simulink model "AirRefueling_Platform_Varyingmass"  (R2023a)
settings: Solver=VariableStepAuto  StartTime=0.0  StopTime=100  FixedStep=0.01  RelTol=1e-3  EnableMultiTasking=on
InitFcn:
  | F16_Init
values from neighbouring files (symbols this model uses):
  A_define = A(1:12,1:12)    [F16_Init.m]
  airSpeed = 393.72    [F16_Init.m]
  alpha0 = trimAlpha*180/pi    (= 6.62393794015)    [F16_Init.m]
  altitude = 9843    [F16_Init.m]
  B_define = A(1:12,13:16)    [F16_Init.m]
  b_ref = 30.0    (= 30)    [F16_Init.m]
  C = [ 1,0,0,zeros(1,15) ... (first row only)    [F16_Init.m]
  C2m = [C(1,:) ... (first row only)    [F16_Init.m]
  C_la = [1,0,zeros(1,4)]    [F16_Init.m]
  C_lon = [1,0,zeros(1,4);0,1,zeros(1,4)]    [F16_Init.m]
  Cdr_ = 0.8    [HoseDrogue_Parameter.m]
  d_f_rc = [3.75;0;-1.75]    [F16_Init.m]
  d_pr_cam = d_pr_rc - d_cam_rc    [F16_Init.m]
  d_pr_rc = [7.6;0.50;-2.44]    [F16_Init.m]
  dLEF = 0    [F16_Init.m]
  dtheta10 = zeros(1,N)    [HoseDrogue_Parameter.m]
  dtheta20 = zeros(1,N)    [HoseDrogue_Parameter.m]
  fi_flag = 1    [F16_Init.m]
  height = 3000    [HoseDrogue_Parameter.m]
  Inertia = [9496,0,-982.0;0,55814.0,0;-982.0,0,63100.0]    [F16_Init.m]
  k_reel = 0.5    [HoseDrogue_Parameter.m]
  Kc = [ ... (first row only)    [F16_Init.m]
  kd = 500    [HoseDrogue_Parameter.m]
  Ki = zeros(4,3)    [F16_Init.m]
  Ki_la = -k_la(:,9)    [F16_Init.m]
  Ki_lon = -k_lon(:,9:10)    [F16_Init.m]
  Kp = zeros(4,18)    [F16_Init.m]
  kp_la = Kp_define(3:4,[2,4,6,9,10,12])    [F16_Init.m]
  kp_lon = Kp_define(1:2,[1,3,5,7,8,11])    [F16_Init.m]
  l0 = (length-l1)/(N-1)    (= 1.44444444444)    [HoseDrogue_Parameter.m]
  l1 = 2    [HoseDrogue_Parameter.m]
  l_density = 4.1    [HoseDrogue_Parameter.m]
  m0 = l0*l_density    (= 5.92222222222)    [HoseDrogue_Parameter.m]
  mass = 636.94    [F16_Init.m]
  Mdr = 29.5    [HoseDrogue_Parameter.m]
  N = 10    [HoseDrogue_Parameter.m]    (also in bsp3.m)
  p0_rc = [-30;1;8]    [F16_Init.m]
  Rdr = 0.305    [HoseDrogue_Parameter.m]
  Rl = 0.0336    [HoseDrogue_Parameter.m]
  T_reel_initial = 1610    [HoseDrogue_Parameter.m]
  theta10 = theta1_100    [HoseDrogue_Parameter.m]
  theta20 = theta2_100    [HoseDrogue_Parameter.m]
  trim_ail = 0.00874607850103852    (= 0.00874607850104)    [F16_Init.m]
  trim_control = [trim_thrust;trim_ele;trim_ail;trim_rud]    [F16_Init.m]
  trim_ele = -2.97973164860638    (= -2.97973164861)    [F16_Init.m]
  trim_rud = 0.0680302158182712    (= 0.0680302158183)    [F16_Init.m]
  trim_state = [0;0;0;0;trimAlpha;0;airSpeed;trimAlpha;0;0;0;0]    [F16_Init.m]
  trim_state1 = [trim_state;0;0;0;0;0;0]    [F16_Init.m]
  trim_thrust = 2279.08519954656    (= 2279.08519955)    [F16_Init.m]
  visual_err = [0.07;0.04;-1.21]    [F16_Init.m]
  vt0 = [120;0;0]    [HoseDrogue_Parameter.m]
undefined symbols (not defined in the file or in its folder): A_la_define, A_lon_define, B_la_define, B_lon_define, CC_la, CC_lon, dockingPoint, F, Light, MIL, STD, v_oil
libraries: aerolibconvert2 x13, etargetslib x11, dspnetwork x10, aerolibasang x8, aerolibatmos2 x3, aerolibobsolete x3, simulink x2, aerolibwind2 x2, aerolibadyn x2, sharedtransform x2, aerolibutil x2, vrlib x1
(part 3 of 4)

== system AirRefueling_Platform_Varyingmass/Receiver system/F16 Nonlinear Model/constant mass model/sec_sys_controller ==
  Pri_Obv_States : Inport
  Sec_Obv_States : Inport  Port=2
  " " : Constant  Value=A_lon_define
  "    " : Constant  Value=B_lon_define
  "     " : Constant  Value=A_la_define
  "      " : Constant  Value=B_la_define
  "    1" : Constant  Value=CC_lon
  "    2" : Constant  Value=CC_la
  Demux : Demux
  Gain1 : Gain  Gain=1000
  Lat_Controller : MATLAB Function  TreatAsAtomicUnit=on
  Lon_Controller : MATLAB Function  TreatAsAtomicUnit=on
  Mux : Mux
  Mux13 : Mux  Inputs=2
  Scope : Scope
  Scope1 : Scope
  TrimState1 : Constant  Value=trim_state
  TrimState2 : Constant  Value=trim_state
  Sec_inputs : Outport  VectorParamsAs1DForOutWhenUnconnected=off
  wires:
  Demux/1 -> Gain1/1
  Gain1/1 -> Mux/1
  Mux/1 -> Sec_inputs/1
  Demux/2 -> Mux/2
  Demux/3 -> Mux/3
  Demux/4 -> Mux/4
  Lon_Controller/2(output) -> Mux13/1
  " "/1 -> Lon_Controller/3(A_lon_define)
  "    "/1 -> Lon_Controller/4(B_lon_define)
  "     "/1 -> Lat_Controller/3(A_la_define)
  "      "/1 -> Lat_Controller/4(B_la_define)
  Lat_Controller/1(output) -> Mux13/2
  "    1"/1 -> Lon_Controller/5(CC_lon)
  "    2"/1 -> Lat_Controller/5(CC_la)
  Lon_Controller/1(s) -> Scope/1
  Lat_Controller/2(s) -> Scope1/1
  Mux13/1 -> Demux/1
  Sec_Obv_States/1 -> Lat_Controller/2(Sec_States), Lon_Controller/1(Sec_States)
  Pri_Obv_States/1 -> Lat_Controller/1(Pri_States), Lon_Controller/2(Pri_States)
  TrimState1/1 -> Lat_Controller/6(trim_states)
  TrimState2/1 -> Lon_Controller/6(trim_states)

== system AirRefueling_Platform_Varyingmass/Receiver system/F16 Nonlinear Model/Variable Mass Model/Aerodynamic Coefficients1/Leading Edge Flap ==
  note: see NASA Technical Paper 1538, p34
  note: Initialize LF_state with -alpha0 value in degrees!!!!
  alpha : Inport
  qbar/ps : Inport  Port=2
  Gain : Gain  Gain=2  SaturateOnIntegerOverflow=on  OutDataTypeStr=Inherit: Same as input  ParamDataTypeStr=Inherit: Same as input
  Gain1 : Gain  Gain=7.25  SaturateOnIntegerOverflow=on  OutDataTypeStr=Inherit: Same as input  ParamDataTypeStr=Inherit: Same as input
  Gain2 : Gain  Gain=1.38  SaturateOnIntegerOverflow=on  OutDataTypeStr=Inherit: Same as input  ParamDataTypeStr=Inherit: Same as input
  LEF Actuator : Subsystem
  LF_state : Integrator  InitialCondition=-alpha0
  Sum : Sum  Inputs=-|+|+  InputSameDT=on  SaturateOnIntegerOverflow=on  OutDataTypeStr=Inherit: Same as first input
  Sum1 : Sum  Inputs=|+-  InputSameDT=on  SaturateOnIntegerOverflow=on  OutDataTypeStr=Inherit: Same as first input
  Sum2 : Sum  Inputs=++|  InputSameDT=on  SaturateOnIntegerOverflow=on  OutDataTypeStr=Inherit: Same as first input
  coeff1 : Constant  Value=1.45
  lef Saturation : Saturate  UpperLimit=25  LowerLimit=0
  r2d6 : Gain  Gain=9.05  SaturateOnIntegerOverflow=on  OutDataTypeStr=Inherit: Same as input  ParamDataTypeStr=Inherit: Same as input
  delta_lef (deg) : Outport
  wires:
  Sum1/1 -> Gain1/1
  Gain1/1 -> LF_state/1
  Gain/1 -> Sum2/1
  Gain2/1 -> Sum/2
  coeff1/1 -> Sum/3
  Sum2/1 -> Sum1/2, Gain2/1
  LF_state/1 -> Sum2/2
  alpha/1 -> Sum1/1, Gain/1
  qbar/ps/1 -> r2d6/1
  r2d6/1 -> Sum/1
  lef Saturation/1 -> delta_lef (deg)/1
  Sum/1 -> LEF Actuator/1(dlef)
  LEF Actuator/1(LEF) -> lef Saturation/1

== system AirRefueling_Platform_Varyingmass/Receiver system/F16 Nonlinear Model/Variable Mass Model/actuator1/Aileron Actuator ==
  delta_a : Inport
  Command Saturation : Saturate  UpperLimit=21.5  LowerLimit=-21.5
  Gain : Gain  Gain=20.2  SaturateOnIntegerOverflow=on  OutDataTypeStr=Inherit: Same as input  ParamDataTypeStr=Inherit: Same as input
  "Integrator " : Integrator  InitialCondition=trim_ail  UpperSaturationLimit=21.5  LowerSaturationLimit=-21.5
  Rate Saturation : Saturate  UpperLimit=80  LowerLimit=-80
  Sum : Sum  Inputs=|+-  InputSameDT=on  SaturateOnIntegerOverflow=on  OutDataTypeStr=Inherit: Same as first input
  ail : Outport
  wires:
  delta_a/1 -> Command Saturation/1
  "Integrator "/1 -> ail/1, Sum/2
  Sum/1 -> Gain/1
  Gain/1 -> Rate Saturation/1
  Command Saturation/1 -> Sum/1
  Rate Saturation/1 -> "Integrator "/1

== system AirRefueling_Platform_Varyingmass/Receiver system/F16 Nonlinear Model/Variable Mass Model/actuator1/Elevator Actuator ==
  delta_e : Inport
  Command Saturation : Saturate  UpperLimit=25  LowerLimit=-25
  Gain : Gain  Gain=20.2  SaturateOnIntegerOverflow=on  OutDataTypeStr=Inherit: Same as input  ParamDataTypeStr=Inherit: Same as input
  "Integrator " : Integrator  InitialCondition=trim_ele  UpperSaturationLimit=25  LowerSaturationLimit=-25
  Rate Saturation : Saturate  UpperLimit=60  LowerLimit=-60
  Sum : Sum  Inputs=|+-  InputSameDT=on  SaturateOnIntegerOverflow=on  OutDataTypeStr=Inherit: Same as first input
  el : Outport
  wires:
  delta_e/1 -> Command Saturation/1
  Command Saturation/1 -> Sum/1
  Sum/1 -> Gain/1
  Gain/1 -> Rate Saturation/1
  "Integrator "/1 -> el/1, Sum/2
  Rate Saturation/1 -> "Integrator "/1

== system AirRefueling_Platform_Varyingmass/Receiver system/F16 Nonlinear Model/Variable Mass Model/actuator1/Rudder Actuator ==
  delta_r : Inport
  Command Saturation : Saturate  UpperLimit=30  LowerLimit=-30
  Gain : Gain  Gain=20.2  SaturateOnIntegerOverflow=on  OutDataTypeStr=Inherit: Same as input  ParamDataTypeStr=Inherit: Same as input
  "Integrator " : Integrator  InitialCondition=trim_rud  UpperSaturationLimit=30  LowerSaturationLimit=-30
  Rate Saturation : Saturate  UpperLimit=120  LowerLimit=-120
  Sum : Sum  Inputs=|+-  InputSameDT=on  SaturateOnIntegerOverflow=on  OutDataTypeStr=Inherit: Same as first input
  rud : Outport
  wires:
  "Integrator "/1 -> rud/1, Sum/2
  Sum/1 -> Gain/1
  delta_r/1 -> Command Saturation/1
  Rate Saturation/1 -> "Integrator "/1
  Gain/1 -> Rate Saturation/1
  Command Saturation/1 -> Sum/1

== system AirRefueling_Platform_Varyingmass/Receiver system/F16 Nonlinear Model/Variable Mass Model/actuator1/Thrust Model ==
  delta_t : Inport
  Command Saturation : Saturate  UpperLimit=19000  LowerLimit=1000
  Gain : Gain  SaturateOnIntegerOverflow=on  OutDataTypeStr=Inherit: Same as input  ParamDataTypeStr=Inherit: Same as input
  "Integrator " : Integrator  InitialCondition=trim_thrust  UpperSaturationLimit=30  LowerSaturationLimit=-30
  Rate Saturation : Saturate  UpperLimit=10000  LowerLimit=-10000
  Sum : Sum  Inputs=|+-  InputSameDT=on  SaturateOnIntegerOverflow=on  OutDataTypeStr=Inherit: Same as first input
  T : Outport
  wires:
  delta_t/1 -> Command Saturation/1
  Gain/1 -> Rate Saturation/1
  "Integrator "/1 -> T/1, Sum/2
  Command Saturation/1 -> Sum/1
  Sum/1 -> Gain/1
  Rate Saturation/1 -> "Integrator "/1

== system AirRefueling_Platform_Varyingmass/Receiver system/F16 Nonlinear Model/constant mass model/F-16/Adding Wind Disturbance ==
  Speed of Sound : Inport
  Air Density : Inport  Port=2
  Wind Velocity : Inport  Port=3  PortDimensions=3
  Wind Angular Rates : Inport  Port=4  PortDimensions=3
  Vb : Inport  Port=5  PortDimensions=3
  p,q,r : Inport  Port=6  PortDimensions=3
  Display : Display
  Dynamic Pressure : aerolibasang/Dynamic Pressure
  "Incidence, Sideslip & Airspeed" : aerolibasang/Incidence, Sideslip, & Airspeed
  Mach Number : aerolibasang/Mach Number
  Mux : Mux  Inputs=2
  Sum : Sum  Inputs=|+-  InputSameDT=on  SaturateOnIntegerOverflow=on  OutDataTypeStr=Inherit: Same as first input
  Sum1 : Sum  Inputs=|++  InputSameDT=on  SaturateOnIntegerOverflow=on  OutDataTypeStr=Inherit: Same as first input
  qbar : Outport  InitialOutput=0
  "p,q,r " : Outport  Port=2
  V : Outport  Port=3
  Mach : Outport  Port=4
  Incid : Outport  Port=5
  wires:
  "Incidence, Sideslip & Airspeed"/3 -> V/1
  Dynamic Pressure/1 -> qbar/1
  Air Density/1 -> Dynamic Pressure/2
  Mach Number/1 -> Mach/1
  Sum/1 -> Dynamic Pressure/1, Mach Number/1, "Incidence, Sideslip & Airspeed"/1
  Vb/1 -> Display/1, Sum/1
  Speed of Sound/1 -> Mach Number/2
  Wind Velocity/1 -> Sum/2
  "Incidence, Sideslip & Airspeed"/2 -> Mux/2  "Beta"
  Mux/1 -> Incid/1
  "Incidence, Sideslip & Airspeed"/1 -> Mux/1  "Alpha"
  p,q,r/1 -> Sum1/1
  Wind Angular Rates/1 -> Sum1/2
  Sum1/1 -> "p,q,r "/1

== system AirRefueling_Platform_Varyingmass/Receiver system/F16 Nonlinear Model/constant mass model/F-16/Aerodynamic Coefficients ==
  Actuators : Inport
  Incid : Inport  Port=2
  Mach : Inport  Port=3
  V : Inport  Port=4
  p,q,r : Inport  Port=5
  qbar/ps : Inport  Port=6
  Angle Conversion : aerolibconvert2/Angle Conversion  IU=rad  OU=deg
  Display : Display
  Interpreted MATLAB Function : MATLABFcn  MATLABFcn=F16Coef1  OutputDimensions=6
  Leading Edge Flap : Subsystem
  Mux : Mux  Inputs=6
  Terminator2 : Terminator
  alpha : Selector  InputPortWidth=2  IndexOptions=Index vector (dialog)  Indices=1  OutputSizes=1
  flag : Constant  Value=fi_flag
  Coeff : Outport  InitialOutput=0
  wires:
  Angle Conversion/1 -> alpha/1, Mux/2
  Incid/1 -> Angle Conversion/1
  qbar/ps/1 -> Leading Edge Flap/2(qbar/ps)
  alpha/1 -> Leading Edge Flap/1(alpha)
  V/1 -> Display/1, Mux/1
  p,q,r/1 -> Mux/3
  Actuators/1 -> Mux/4
  flag/1 -> Mux/5
  Mach/1 -> Terminator2/1
  Interpreted MATLAB Function/1 -> Coeff/1
  Mux/1 -> Interpreted MATLAB Function/1
  Leading Edge Flap/1(delta_lef (deg)) -> Mux/6

== system AirRefueling_Platform_Varyingmass/Receiver system/F16 Nonlinear Model/constant mass model/F-16/Environment Models ==
  Xe : Inport  PortDimensions=3
  DCM : Inport  Port=2
  COESA Atmosphere Model : aerolibatmos2/COESA Atmosphere Model  units=English (Velocity in ft/s)  spec=1976 COESA-extended U.S. Standard Atmosphere  model=Profile  profile_var=High temperature  profile_percent=10%  profile_alt=5 km (16404 ft)  envelope_var=High temperature  envelope_percent=1%  action=None
  Display : Display
  Display1 : Display
  Gravity in Earth Axes : Gain  Gain=mass  SaturateOnIntegerOverflow=on  OutDataTypeStr=Inherit: Same as input  ParamDataTypeStr=Inherit: Same as input
  Height : Selector  InputPortWidth=3  IndexOptions=Index vector (dialog)  Indices=[3]  OutputSizes=1
  Inertial to Body : Product  Multiplication=Matrix(*)  InputSameDT=on  SaturateOnIntegerOverflow=on  OutDataTypeStr=Inherit: Same as first input
  Latitude : Constant  Value=0
  Mux : Mux  Inputs=3
  Product6 : Product  Inputs=**  InputSameDT=on  SaturateOnIntegerOverflow=on  OutDataTypeStr=Inherit: Same as first input
  Reshape : Reshape
  Terminator : Terminator
  "WGS84 Gravity Model " : aerolibobsolete/WGS84 Gravity Model   model=WGS84 Taylor Series  units=English  no_atmos=on  precessing=on  jd_loc=off  month=October  day=10  year=2004  no_centrifugal=on  action=None
  r2d5 : Gain  Gain=1715  SaturateOnIntegerOverflow=on  OutDataTypeStr=Inherit: Same as input  ParamDataTypeStr=Inherit: Same as input
  z-->h : Abs
  Fg : Outport  InitialOutput=0
  Speed of Sound : Outport  Port=2  InitialOutput=0
  Air Density : Outport  Port=3  InitialOutput=0
  PS : Outport  Port=4
  wires:
  Reshape/1 -> Inertial to Body/2
  Mux/1 -> "WGS84 Gravity Model "/1
  z-->h/1 -> Mux/3, COESA Atmosphere Model/1
  COESA Atmosphere Model/2 -> Speed of Sound/1
  COESA Atmosphere Model/3 -> Terminator/1
  Height/1 -> z-->h/1
  Xe/1 -> Height/1
  Latitude/1 -> Mux/2, Mux/1
  "WGS84 Gravity Model "/1 -> Gravity in Earth Axes/1
  Gravity in Earth Axes/1 -> Reshape/1
  DCM/1 -> Inertial to Body/1
  Inertial to Body/1 -> Display1/1, Fg/1
  COESA Atmosphere Model/4 -> Product6/2, Air Density/1
  COESA Atmosphere Model/1 -> r2d5/1
  Product6/1 -> Display/1, PS/1
  r2d5/1 -> Product6/1

== system AirRefueling_Platform_Varyingmass/Receiver system/F16 Nonlinear Model/constant mass model/F-16/Forces and Moments ==
  Coeff : Inport
  Thrust : Inport  Port=2
  qbar : Inport  Port=3
  "Aerodynamic Forces and Moments " : aerolibadyn/Aerodynamic Forces and Moments   inputAxes=Body  outputForceAxes=Body  outputMomentAxes=Body  S=S_ref  b=b_ref  cbar=d_ref
  Center of Gravity : Constant  Value=[-0 0 0]
  Center of Pressure : Constant  Value=[-0 0 0]
  Sum : Sum  Inputs=++|  InputSameDT=on  SaturateOnIntegerOverflow=on  OutDataTypeStr=Inherit: Same as first input
  X,Y,Z : Outport  InitialOutput=0
  LMN : Outport  Port=2  InitialOutput=0
  wires:
  Center of Pressure/1 -> "Aerodynamic Forces and Moments "/4
  Center of Gravity/1 -> "Aerodynamic Forces and Moments "/3
  "Aerodynamic Forces and Moments "/1 -> Sum/2
  "Aerodynamic Forces and Moments "/2 -> LMN/1
  Sum/1 -> X,Y,Z/1
  Thrust/1 -> Sum/1
  qbar/1 -> "Aerodynamic Forces and Moments "/2
  Coeff/1 -> "Aerodynamic Forces and Moments "/1

== system AirRefueling_Platform_Varyingmass/Receiver system/F16 Nonlinear Model/constant mass model/F-16/Subsystem ==
  <Eular(rad)> : Inport
  DCM : Inport  Port=2
  Ve : Inport  Port=3
  X_relative : Inport  Port=4
  pqr : Inport  Port=5
  Constant1 : Constant  Value=mass
  Constant5 : Constant  Value=dockingPoint
  Direction Cosine Matrix to Quaternions : sharedtransform/Direction Cosine Matrix  to Quaternions  aMode=aMode  action=None  tolerance=eps(2)
  Direction Cosine Matrix to Quaternions1 : sharedtransform/Direction Cosine Matrix  to Quaternions  aMode=aMode  action=None  tolerance=eps(2)
  Euler to DCM : aerolibtransform2/Wind Angles to  Direction Cosine Matrix
  Ground Model : MATLAB Function  TreatAsAtomicUnit=on
  Length Conversion : aerolibconvert2/Length Conversion  IU=ft  OU=m
  OnGroundFaceup : MATLAB Function  TreatAsAtomicUnit=on
  Product1 : Product  Multiplication=Matrix(*)
  Quaternion Inverse : aerolibutil/Quaternion Inverse
  Quaternion Multiplication : aerolibutil/Quaternion Multiplication
  Scope : Scope
  Scope1 : Scope
  Scope2 : Scope
  Sum : Sum  Inputs=|-+
  F1 : Outport
  M1 : Outport  Port=2
  wires:
  Length Conversion/1 -> Sum/1, Ground Model/3(X_relative)
  Direction Cosine Matrix to Quaternions/1 -> Quaternion Multiplication/2
  Constant5/1 -> Sum/2, Ground Model/6(dockingPoint)
  pqr/1 -> Ground Model/2(wb)
  Euler to DCM/1 -> Direction Cosine Matrix to Quaternions1/1
  DCM/1 -> Product1/1, Direction Cosine Matrix to Quaternions/1
  Ground Model/1(F1) -> Scope/1, Product1/2
  Quaternion Inverse/1 -> Quaternion Multiplication/1
  <Eular(rad)>/1 -> OnGroundFaceup/1(EulerAng)
  OnGroundFaceup/1(y) -> Euler to DCM/1
  X_relative/1 -> Length Conversion/1
  Direction Cosine Matrix to Quaternions1/1 -> Quaternion Inverse/1
  Product1/1 -> Scope1/1, F1/1
  Quaternion Multiplication/1 -> Ground Model/5(Quet)
  Ground Model/2(M1) -> M1/1
  Ve/1 -> Ground Model/4(Ve)
  Sum/1 -> Scope2/1
  Constant1/1 -> Ground Model/1(mass)

== system AirRefueling_Platform_Varyingmass/Receiver system/F16 Nonlinear Model/constant mass model/F-16/actuator ==
  u : Inport
  Aileron Actuator : Subsystem
  Demux : Demux
  Elevator Actuator : Subsystem
  Mux : Mux
  Mux1 : Mux  Inputs=3
  Mux2 : Mux  Inputs=3
  Rudder Actuator : Subsystem
  Thrust Model : Subsystem
  Ty : Constant  Value=0
  Tz : Constant  Value=0
  Ang : Outport
  T : Outport  Port=2
  uc : Outport  Port=3
  wires:
  u/1 -> Demux/1
  Mux2/1 -> Ang/1
  Thrust Model/1(T) -> Mux/1, Mux1/1  "Tx"
  Ty/1 -> Mux1/2
  Tz/1 -> Mux1/3
  Mux1/1 -> T/1
  Mux/1 -> uc/1
  Demux/1 -> Thrust Model/1(delta_t)
  Elevator Actuator/1(el) -> Mux2/1, Mux/2  "el"
  Aileron Actuator/1(ail) -> Mux2/2, Mux/3  "ail"
  Rudder Actuator/1(rud) -> Mux2/3, Mux/4  "rud"
  Demux/2 -> Elevator Actuator/1(delta_e)
  Demux/3 -> Aileron Actuator/1(delta_a)
  Demux/4 -> Rudder Actuator/1(delta_r)

== system AirRefueling_Platform_Varyingmass/Receiver system/F16 Nonlinear Model/Variable Mass Model/Aerodynamic Coefficients1/Leading Edge Flap/LEF Actuator ==
  dlef : Inport
  Command Saturation : Saturate  UpperLimit=25  LowerLimit=0
  Gain3 : Gain  Gain=1/0.136  SaturateOnIntegerOverflow=on  OutDataTypeStr=Inherit: Same as input  ParamDataTypeStr=Inherit: Same as input
  "Integrator " : Integrator  InitialCondition=dLEF  UpperSaturationLimit=21.5  LowerSaturationLimit=-21.5
  Rate Saturation : Saturate  UpperLimit=25  LowerLimit=-25
  Sum3 : Sum  Inputs=|+-  InputSameDT=on  SaturateOnIntegerOverflow=on  OutDataTypeStr=Inherit: Same as first input
  LEF : Outport
  wires:
  Gain3/1 -> Rate Saturation/1
  Rate Saturation/1 -> "Integrator "/1
  "Integrator "/1 -> LEF/1, Sum3/2
  Sum3/1 -> Gain3/1
  dlef/1 -> Command Saturation/1
  Command Saturation/1 -> Sum3/1

== system AirRefueling_Platform_Varyingmass/Receiver system/F16 Nonlinear Model/constant mass model/F-16/Aerodynamic Coefficients/Leading Edge Flap ==
  note: see NASA Technical Paper 1538, p34
  note: Initialize LF_state with -alpha0 value in degrees!!!!
  alpha : Inport
  qbar/ps : Inport  Port=2
  Gain : Gain  Gain=2  SaturateOnIntegerOverflow=on  OutDataTypeStr=Inherit: Same as input  ParamDataTypeStr=Inherit: Same as input
  Gain1 : Gain  Gain=7.25  SaturateOnIntegerOverflow=on  OutDataTypeStr=Inherit: Same as input  ParamDataTypeStr=Inherit: Same as input
  Gain2 : Gain  Gain=1.38  SaturateOnIntegerOverflow=on  OutDataTypeStr=Inherit: Same as input  ParamDataTypeStr=Inherit: Same as input
  LEF Actuator : Subsystem
  LF_state : Integrator  InitialCondition=-alpha0
  Sum : Sum  Inputs=-|+|+  InputSameDT=on  SaturateOnIntegerOverflow=on  OutDataTypeStr=Inherit: Same as first input
  Sum1 : Sum  Inputs=|+-  InputSameDT=on  SaturateOnIntegerOverflow=on  OutDataTypeStr=Inherit: Same as first input
  Sum2 : Sum  Inputs=++|  InputSameDT=on  SaturateOnIntegerOverflow=on  OutDataTypeStr=Inherit: Same as first input
  coeff1 : Constant  Value=1.45
  lef Saturation : Saturate  UpperLimit=25  LowerLimit=0
  r2d6 : Gain  Gain=9.05  SaturateOnIntegerOverflow=on  OutDataTypeStr=Inherit: Same as input  ParamDataTypeStr=Inherit: Same as input
  delta_lef (deg) : Outport
  wires:
  Sum1/1 -> Gain1/1
  Gain1/1 -> LF_state/1
  Gain/1 -> Sum2/1
  Gain2/1 -> Sum/2
  coeff1/1 -> Sum/3
  Sum2/1 -> Sum1/2, Gain2/1
  LF_state/1 -> Sum2/2
  alpha/1 -> Sum1/1, Gain/1
  qbar/ps/1 -> r2d6/1
  r2d6/1 -> Sum/1
  lef Saturation/1 -> delta_lef (deg)/1
  Sum/1 -> LEF Actuator/1(dlef)
  LEF Actuator/1(LEF) -> lef Saturation/1

== system AirRefueling_Platform_Varyingmass/Receiver system/F16 Nonlinear Model/constant mass model/F-16/actuator/Aileron Actuator ==
  delta_a : Inport
  Command Saturation : Saturate  UpperLimit=21.5  LowerLimit=-21.5
  Gain : Gain  Gain=20.2  SaturateOnIntegerOverflow=on  OutDataTypeStr=Inherit: Same as input  ParamDataTypeStr=Inherit: Same as input
  "Integrator " : Integrator  InitialCondition=trim_ail  UpperSaturationLimit=21.5  LowerSaturationLimit=-21.5
  Rate Saturation : Saturate  UpperLimit=80  LowerLimit=-80
  Sum : Sum  Inputs=|+-  InputSameDT=on  SaturateOnIntegerOverflow=on  OutDataTypeStr=Inherit: Same as first input
  ail : Outport
  wires:
  delta_a/1 -> Command Saturation/1
  "Integrator "/1 -> ail/1, Sum/2
  Sum/1 -> Gain/1
  Gain/1 -> Rate Saturation/1
  Command Saturation/1 -> Sum/1
  Rate Saturation/1 -> "Integrator "/1

== system AirRefueling_Platform_Varyingmass/Receiver system/F16 Nonlinear Model/constant mass model/F-16/actuator/Elevator Actuator ==
  delta_e : Inport
  Command Saturation : Saturate  UpperLimit=25  LowerLimit=-25
  Gain : Gain  Gain=20.2  SaturateOnIntegerOverflow=on  OutDataTypeStr=Inherit: Same as input  ParamDataTypeStr=Inherit: Same as input
  "Integrator " : Integrator  InitialCondition=trim_ele  UpperSaturationLimit=25  LowerSaturationLimit=-25
  Rate Saturation : Saturate  UpperLimit=60  LowerLimit=-60
  Sum : Sum  Inputs=|+-  InputSameDT=on  SaturateOnIntegerOverflow=on  OutDataTypeStr=Inherit: Same as first input
  el : Outport
  wires:
  delta_e/1 -> Command Saturation/1
  Command Saturation/1 -> Sum/1
  Sum/1 -> Gain/1
  Gain/1 -> Rate Saturation/1
  "Integrator "/1 -> el/1, Sum/2
  Rate Saturation/1 -> "Integrator "/1

== system AirRefueling_Platform_Varyingmass/Receiver system/F16 Nonlinear Model/constant mass model/F-16/actuator/Rudder Actuator ==
  delta_r : Inport
  Command Saturation : Saturate  UpperLimit=30  LowerLimit=-30
  Gain : Gain  Gain=20.2  SaturateOnIntegerOverflow=on  OutDataTypeStr=Inherit: Same as input  ParamDataTypeStr=Inherit: Same as input
  "Integrator " : Integrator  InitialCondition=trim_rud  UpperSaturationLimit=30  LowerSaturationLimit=-30
  Rate Saturation : Saturate  UpperLimit=120  LowerLimit=-120
  Sum : Sum  Inputs=|+-  InputSameDT=on  SaturateOnIntegerOverflow=on  OutDataTypeStr=Inherit: Same as first input
  rud : Outport
  wires:
  "Integrator "/1 -> rud/1, Sum/2
  Sum/1 -> Gain/1
  delta_r/1 -> Command Saturation/1
  Rate Saturation/1 -> "Integrator "/1
  Gain/1 -> Rate Saturation/1
  Command Saturation/1 -> Sum/1

== system AirRefueling_Platform_Varyingmass/Receiver system/F16 Nonlinear Model/constant mass model/F-16/actuator/Thrust Model ==
  delta_t : Inport
  Command Saturation : Saturate  UpperLimit=19000  LowerLimit=1000
  Gain : Gain  SaturateOnIntegerOverflow=on  OutDataTypeStr=Inherit: Same as input  ParamDataTypeStr=Inherit: Same as input
  "Integrator " : Integrator  InitialCondition=trim_thrust  UpperSaturationLimit=30  LowerSaturationLimit=-30
  Rate Saturation : Saturate  UpperLimit=10000  LowerLimit=-10000
  Sum : Sum  Inputs=|+-  InputSameDT=on  SaturateOnIntegerOverflow=on  OutDataTypeStr=Inherit: Same as first input
  T : Outport
  wires:
  delta_t/1 -> Command Saturation/1
  Gain/1 -> Rate Saturation/1
  "Integrator "/1 -> T/1, Sum/2
  Command Saturation/1 -> Sum/1
  Sum/1 -> Gain/1
  Rate Saturation/1 -> "Integrator "/1

== system AirRefueling_Platform_Varyingmass/Receiver system/F16 Nonlinear Model/constant mass model/F-16/Aerodynamic Coefficients/Leading Edge Flap/LEF Actuator ==
  dlef : Inport
  Command Saturation : Saturate  UpperLimit=25  LowerLimit=0
  Gain3 : Gain  Gain=1/0.136  SaturateOnIntegerOverflow=on  OutDataTypeStr=Inherit: Same as input  ParamDataTypeStr=Inherit: Same as input
  "Integrator " : Integrator  InitialCondition=dLEF  UpperSaturationLimit=21.5  LowerSaturationLimit=-21.5
  Rate Saturation : Saturate  UpperLimit=25  LowerLimit=-25
  Sum3 : Sum  Inputs=|+-  InputSameDT=on  SaturateOnIntegerOverflow=on  OutDataTypeStr=Inherit: Same as first input
  LEF : Outport
  wires:
  Gain3/1 -> Rate Saturation/1
  Rate Saturation/1 -> "Integrator "/1
  "Integrator "/1 -> LEF/1, Sum3/2
  Sum3/1 -> Gain3/1
  dlef/1 -> Command Saturation/1
  Command Saturation/1 -> Sum3/1

== matlab function AirRefueling_Platform_Varyingmass/SimToVR2 ==
  data: PosPr1 input; PosTb1 input; y output
function y = SimToVR(PosPr1,PosTb1)
%#codegen

%%函数名：SimToVR
%%用途  ：将软管锥套坐标输出转换为VR输入
%%输入  ：PosPr - 受油机椎管坐标， PlsTb - 软管坐标数据
%%输出  ：VrPos - 软管和受油机VR位置，VrAngle - 旋转角度输出
%%作者  ：戴训华
%%时间  ：2014/3/19

PosPr = PosPr1(1:3);
AttitudeRecei = [0;-0;0+0.115609];

PosTb = PosTb1(1:60);

VrAngle = zeros(22*4,1);
VrPos = zeros(22*3,1);


for j = 1:21                        %前20为软管坐标数据，后1为软管平滑过渡处理
    if j == 1
        pX = [0, 0, 0]';            %软管起点
        pY = PosTb(3*j-2:3*j);      %软杆终点
    elseif j == 21                  %多加一段杆，做过渡
        pX = PosTb(3*j-5:3*j-3);
        pY = [PosTb(3*j-5)-0.7163*cos(8/180*pi),PosTb(3*j-4),PosTb(3*j-3)+0.7163*sin(8/180*pi)]'+[0;-0.2;0];
    else
        pX = PosTb(3*j-5:3*j-3);
        pY = PosTb(3*j-2:3*j); 
    end
    
    pZ = (pX + pY)/2;               %中点坐标
    pZ = pZ * 8/3;                  %到VR中比例的缩放

    vAxis = [0,0,-1]';               %水平轴
    vTb = pY - pX;                  %杆的方向
    
    axis1 = null([vAxis';vTb']);%获取垂直向量
    vRot = axis1(:,1)';             %得到旋转轴
    
    if vRot(2) < 0
        vRot = -vRot;
    end
    
    VrAngle(4*j-3:4*j-1) = [vRot(1),vRot(3),vRot(2)]';
    VrAngle(4*j) = acos(vAxis'*vTb / sqrt(vAxis'*vAxis * vTb'*vTb));
    
    VrPos(3*j-2:3*j) = [pZ(1),-pZ(3),pZ(2)]';
end
%y = u;
VrAngle(81:84)=VrAngle(81:84)+[0.2714;0;0;0]; %微调锥套姿态
VrPos(61:63)=VrPos(61:63)+[0;0.00;0.25];      %微调锥套位置

VrAngle(85:88)=[AttitudeRecei(1);AttitudeRecei(2);AttitudeRecei(3);norm(AttitudeRecei)];
pZ = PosPr+[0 0-0.1 0-0.1]';
pZ = pZ * 8/3;
VrPos(3*22-2:3*22) = [pZ(1),-pZ(3),pZ(2)]';

y = [VrAngle;VrPos];

== matlab function AirRefueling_Platform_Varyingmass/Hose-drogue system/DRdynamics/HDU/MATLAB Function2 ==
  data: l_1 input; T0 input; Tt output size=1; t input; dl input; l1 parameter; k_reel parameter; kd parameter
function Tt = fcn(l_1,T0,t,dl, l1,k_reel,kd)
Treel = T0*(l_1/l1)^k_reel;
Tt = t - Treel - kd*dl;

== matlab function AirRefueling_Platform_Varyingmass/Receiver system/F16 Nonlinear Model/constant mass model/Observer/Nonlinear Term ==
  data: trimed_states input; y output; A_la_define input; A_lon_define input; trim_states input
function y = fcn(trimed_states,A_la_define,A_lon_define,trim_states)
%% 原状态值（配平前的）
ori_states = trimed_states + trim_states;
phi_ori = ori_states(4);
theta_ori = ori_states(5);
psi_ori = ori_states(6);
Vr_ori = ori_states(7);
alpha_ori = ori_states(8);
beta_ori = ori_states(9);
p_ori = ori_states(10);
q_ori = ori_states(11);
r_ori = ori_states(12);

ug_ori = Vr_ori * cos(alpha_ori) * cos(beta_ori);
vg_ori = Vr_ori * sin(beta_ori);
wg_ori = Vr_ori * sin(alpha_ori) * cos(beta_ori);

xg_ori = ug_ori*cos(theta_ori)*cos(psi_ori) + vg_ori*(sin(phi_ori)*sin(theta_ori)*cos(psi_ori)-cos(phi_ori)*sin(psi_ori)) ...
     + wg_ori*(sin(phi_ori)*sin(psi_ori)+cos(phi_ori)*sin(theta_ori)*cos(psi_ori));
yg_ori = ug_ori*cos(theta_ori)*sin(psi_ori) + vg_ori*(sin(phi_ori)*sin(theta_ori)*sin(psi_ori)+cos(phi_ori)*cos(psi_ori)) ...
     + wg_ori*(-sin(phi_ori)*cos(psi_ori) + cos(phi_ori)*sin(theta_ori)*sin(psi_ori));
hg_ori = ug_ori*sin(theta_ori) - vg_ori*sin(phi_ori)*cos(theta_ori) - wg_ori*cos(phi_ori)*cos(theta_ori);
%% 差状态值（配平后的）
phi_trimed = trimed_states(4);
theta_trimed = trimed_states(5);
psi_trimed = trimed_states(6);
Vr_trimed = trimed_states(7);
alpha_trimed = trimed_states(8);
beta_trimed = trimed_states(9);
p_trimed = trimed_states(10);
q_trimed = trimed_states(11);
r_trimed = trimed_states(12);

% x_nonlinear = Vr_ori * cos(theta_ori - alpha_ori) - A_lon_define(1,3) * theta_trimed - Vr_ori;
% y_nonlinear = Vr_ori * cos(theta_ori - alpha_ori) * sin(psi_ori + beta_ori) - A_la_define(1,2) * phi_trimed - A_la_define(1,3) * psi_trimed - A_la_define(1,4) * beta_trimed;
% h_nonlinear = hg_ori  - A_lon_define(2,3) * (theta_trimed - alpha_trimed);

x_nonlinear = Vr_ori * cos(theta_ori - alpha_ori) - trim_states(7)*cos(trim_states(5)-trim_states(8)) - A_lon_define(1,3) * theta_trimed - Vr_trimed;
y_nonlinear = yg_ori - A_la_define(1,2) * phi_trimed - A_la_define(1,3) * psi_trimed - A_la_define(1,4) * beta_trimed;
h_nonlinear = Vr_ori * sin(theta_ori - alpha_ori) - A_lon_define(2,3) * (theta_trimed - alpha_trimed);
psi_nonlinear = (q_ori*sin(phi_ori) + r_ori*cos(phi_ori))/cos(theta_ori) - A_la_define(3,6) * r_trimed;  % psi
phi_nonlinear = p_ori + tan(theta_ori)*(q_ori*sin(phi_ori)+r_ori*cos(phi_ori)) - A_la_define(2,5) * p_trimed - A_la_define(2,6) * r_trimed;  % phi


y = [x_nonlinear; y_nonlinear; h_nonlinear; phi_nonlinear; 0; psi_nonlinear; 0;0;0;0;0;0];

== matlab function AirRefueling_Platform_Varyingmass/SimToUE ==
  data: y output; PosRc input; PosTb1 input; Pos_dr2tx output
function [y,Pos_dr2tx] = SimToVR(PosRc,PosTb1)
%#codegen

%%函数名：SimToVR
%%用途  ：将软管锥套坐标输出转换为VR输入
%%输入  ：PosPr - 受油机坐标， PlsTb - 软管坐标数据
%%输出  ：VrPos - 软管和受油机VR位置，VrAngle - 旋转角度输出
%%作者  ：戴训华
%%时间  ：2014/3/19

Pos_rc2tx = PosRc(4:6);
% add PosPr1(4:6)存储的是受油机的姿态  模型中在输出姿态[phi, theta, psai]后加上了trim_state1=[0;0.1156,0],这里又给减掉了
% 无人机先绕机体系 z 轴旋转 ψ \psiψ，再绕机体系 y 轴旋转 θ \thetaθ，最后绕机体系 x 轴旋转 ϕ \phiϕ，[yaw,pitch,roll]
% AttitudeRecei = [PosPr1(4);-PosPr1(6);PosPr1(5)-0.115609];
AttitudeRecei = [0;0.1156;0];
PosTb = PosTb1(1:60);

% 这个不用 用的是通过最后一根杆子生成锥套的方法
PosDr = PosTb1(61:63);

% 这里是20根软管+1个锥套+1个受油机 
VrAngle = zeros(22*3,1);
VrPos = zeros(22*3,1);

% 对于发送模型的视觉修正  全部在这里
% 由于这里只管发送 所以必须让前面模型在计算时也考虑这些修正，这样才能把各种计算都对上
hose_delta_pos = [0;0;0];                      % 视觉对齐 让软管都上升1m
drogue_delta_pos =[0;0;.04];                   % 调整锥套的位置 让它和最后一根软管对上 和软管一样先调整1m，再微调 其实就是 hose_delta_pos + [0.85;0;-0.15]
drogue_delta_angle = [0;0;0];                  % 调整锥套的角度 让它和最后一根软管的角度切合 rpy，pitch向上是正向下是负 [0;-8/180*pi;pi]
drogue_visual_pos = [-0.05;0;1.1];             % 这里要将锥套的位置反馈给前面做计算，要将锥套的视觉位置dr2tx+drogue_visual_pos=实际的锥套位置  
                                               % 方法是通过视觉识别得到的dr2cam(z)+cam2rc(z)+dr2tx(z)=rc2tx(z).这里dr2cam是准确的，只有dr2tx可变，所以修正到这里

% add
scale = 1;
for j = 1:21                        %前20为软管坐标数据，后1为软管平滑过渡处理
    if j == 1
        pX = [0, 0, 0]';            %软管起点
        pY = PosTb(3*j-2:3*j);      %软杆终点
                                    % 不用平滑的 直接用锥套的真实位置
    elseif j == 21                  %多加一段杆，做过渡
        pX = PosTb(3*j-5:3*j-3);
        pY = [PosTb(3*j-5)-0.7163*cos(8/180*pi),PosTb(3*j-4),PosTb(3*j-3)+0.7163*sin(8/180*pi)]';
    else
        pX = PosTb(3*j-5:3*j-3);
        pY = PosTb(3*j-2:3*j); 
    end
    
    pZ = (pX + pY)/2;                   %中点坐标

    %到VR中比例的缩放
    pZ = pZ * scale;
    
    vAxis = [0,0,-1]';                  %水平轴
    vTb = pY - pX;                      %杆的方向
    
    axis1 = null([vAxis';vTb']);        %获取垂直向量
    vRot = axis1(:,1)';                 %得到旋转轴
    
    if vRot(2) < 0
        vRot = -vRot;
    end
 
    yaw_xoz = asin(vTb(2) / sqrt(vTb(1)*vTb(1) + vTb(2)*vTb(2)+ vTb(3)*vTb(3)));
    pitch_z = pi - atan(vTb(3) / vTb(1));
%     pitch_z = atan(vTb(3) / vTb(1));
    roll = 0;   % 圆柱形hose，不用计算roll   
    VrAngle(3*j-2:3*j) = [yaw_xoz, pitch_z, roll];
    % 视觉对齐 让软管都上升hose_delta_posm
    VrPos(3*j-2:3*j) = [pZ(1);pZ(2);pZ(3)] + hose_delta_pos;
end
% add 发送的是受油机的位置
VrAngle(64:66)=[AttitudeRecei(1);AttitudeRecei(2);AttitudeRecei(3)];

pZ = Pos_rc2tx;
pZ = pZ * scale;
VrPos(3*22-2:3*22) = [pZ(1),pZ(2),pZ(3)]';


tmp1 = VrPos(1:60,:);                               % 软管位置
tmp2 = VrPos(61:63,:) + drogue_delta_pos;           % 锥套位置
tmp3 = VrPos(64:66,:) ;                             % 受油机位置 
tmp4 = VrAngle(1:60,:);                             % 软管角度
tmp5 = tmp4(58:60) + drogue_delta_angle;            % 锥套角度 使用的是最后一根软管的角度
tmp6 = VrAngle(64:66,:);                            % 受油机角度

tmp=[tmp1;tmp4;tmp2;tmp5;tmp3;tmp6];
y = tmp;

% 发送反馈给前面的锥套位置由于视觉上有差异，所以需要修正 但是实际上发送的是tmp2，并没有发送调整过的值 
Pos_dr2tx=tmp2+drogue_visual_pos;

== matlab function AirRefueling_Platform_Varyingmass/Tanker system/   ==
  data: u input; y output
function y = WindTurFromTank(u)
%#codegen

y = TankerVortexWindField(u);

== matlab function AirRefueling_Platform_Varyingmass/Hose-drogue system/DRdynamics/Hose-Drogue1/Calculate the Acceleration of the Links1/MATLAB Function2 ==
  data: t0 output size=1; T input; q input; t output
function [t0,t] = fcn(T,q)
% 由于编译报错所以用下面两行来替换第三行。
t = zeros(10,1);
t = inv(T)*q;
% t = T\q;
t0 = t(1);

== matlab function AirRefueling_Platform_Varyingmass/Hose-drogue system/DRdynamics/Hose-Drogue1/Calculate the Acceleration of the Links1/MATLAB Function3 ==
  data: t input; Q input; n input; m1 input; Mdr input; a output; N parameter; m0 parameter
function a = fcn(t,Q,n,m1,Mdr, N,m0)
a = zeros(3,N);
a(:,1) = (t(1)*n(:,1) - t(2)*n(:,2) + Q(:,1))/m1;
for i = 2:N-1
    a(:,i) = (t(i)*n(:,i) - t(i+1)*n(:,i+1) + Q(:,i))/m0;
end
a(:,N) = (t(N)*n(:,N) + Q(:,N))/(m0/2 + Mdr);                %注意最后一个节点的质量！！

== matlab function AirRefueling_Platform_Varyingmass/Hose-drogue system/DRdynamics/Hose-Drogue1/Calculate the Acceleration of the Links1/MATLAB Function4 ==
  data: n input; dn input; q output; Q input; m1 input; l1 input; ddl1 input; a0 input; N parameter; l0 parameter; m0 parameter
function q = fcn(n,dn,Q,m1,l1,ddl1,a0, N,l0,m0)

% n = 连杆的方向向量，想上为正 向量3*N
% Q = 连杆所受的合外力 向量3*N
% m = 连杆质量 向量1*N
% l = 连杆长度 向量1*N
% dl = 连杆长度的一阶导数 向量1*N
% ddl = 连杆长度的二阶导数 向量1*N
% a0 = 连接点的加速度 向量3*1

%%%%求张力t%%%%%%%%%%%%%%%%%%%%%%%%%%%%%%%%%%%%%%%%%%%%%%%%%%%%%%
q = zeros(N,1);
q(1,1) = m1*l1*dn(:,1)'*dn(:,1) - Q(:,1)'*n(:,1) + m1*a0'*n(:,1) - m1*ddl1;
q(2,1) = l0*dn(:,2)'*dn(:,2) + (1/m1*Q(:,1) - 1/m0*Q(:,2))'*n(:,2); % 可参考有关变长度连杆的《推导》
for i = 3:N
    q(i,1) = l0*dn(:,i)'*dn(:,i) + (1/m0*Q(:,i-1) - 1/m0*Q(:,i))'*n(:,i);
end

== matlab function AirRefueling_Platform_Varyingmass/Receiver system/F16 Nonlinear Model/constant mass model/F-16/Subsystem/Ground Model ==
  settings: updateMethod=DISCRETE
  data: mass input; wb input; X_relative input; F1 output; Ve input; M1 output; Quet input; dockingPoint input
function [F1,M1] = fcn(mass,wb,X_relative,Ve,Quet,dockingPoint)
% This is a ground model that can provides reaction force and reaction torque
% 受油机飞行过的距离大约为[7.473，-1.639，-0.8798]时，能够对准
% 此时椎管估计值-真实值=[0.1107，0.008，0.05]
%  这里将锥套中的空间深度=半径=0.35m 那么方程就是z^2+y^2-(0.35-x)^2=0
%  那么xyz如果在空间内部带进去算出来的右边值小于等于0
F1=[0;0;0];
M1=[0;0;0];
x=X_relative(1)-dockingPoint(1);
y=X_relative(2)-dockingPoint(2);
z=X_relative(3)-dockingPoint(3);


if x>=-0.35 && x<=0.2
    % 当x进入一定范围之内时，才能计算误差
    % 当前位置减去定点的位置 相当于把定点放在了原点 x^2 = y^2 + z^2 
    % 分成xyz三个方向进行误差计算 
    % x的范围[-0.2,0.45]  yz的范围相同,就是x一定时，半径时y=z=x对应的圆形的范围[-y,y]
    % 给定了x之后 要判断两个 第一个是在这个圆形范围内，第二个是距离圆心的距
    error =z^2+y^2-x^2; 
    if  error < 0
        % x方向的力
        % 0- -0.2m 戳出去了
        if x<-0.25
           F1(1)=-mass*Ve(1);
        % 0.1-0m
        elseif x>-0.25 && x<0.1
            F1(1)=-5*mass*Ve(1); 
        % 0.1m以上
        else
            F1(1)=-10*mass*Ve(1); 
        end
        
        % y方向的力
        % 椎管位置在圆心的右边 且和做边沿相距0.1*x 且速度还是向右时，给一个大的斥力
        if y>0 && abs(y)>0.9*abs(x) && Ve(2)>0
            F1(2)=-10*mass*Ve(2);          
        end
        % 椎管位置在圆心的右边 且和做边沿相距0.1*x，给一个大的斥力
        if y<0 && abs(y)>0.9*abs(x)&& Ve(2)<0
            F1(2)=-10*mass*Ve(2);          
        end
        
        % z方向的力
        % 椎管在锥套中心上方 要让飞机往下 z轴力为正
        if z>0 && abs(z)>0.9*abs(x) && Ve(3)>0
           F1(3)=-10*mass*Ve(3);
        end
        if z<0 && abs(z)>0.9*abs(x) && Ve(3)<0
           F1(3)=-10*mass*Ve(3);
        end
           
        M1=-20*[Quet(2);Quet(3);Quet(4)]-5*wb;
        M1 = M1 *0.0333;
    end
end     

F1=[0;0;0];
M1=[0;0;0];

== matlab function AirRefueling_Platform_Varyingmass/Receiver system/F16 Nonlinear Model/constant mass model/F-16/Subsystem/OnGroundFaceup ==
  data: EulerAng input; y output
function y = fcn(EulerAng)

targetRoll = 0;
% if cos(EulerAng(1))<0
%     targetRoll=pi;  
% end

targetPitch = 0;
% if cos(EulerAng(2))<0
%         targetPitch=pi;
% end
    
y = [targetRoll;targetPitch;EulerAng(3)];

== matlab function AirRefueling_Platform_Varyingmass/Hose-drogue system/Collision Detection/MATLAB Function1 ==
  settings: updateMethod=DISCRETE
  data: Pos_pr input; F output; V_pr input; Pos_dr input; V_dr input; Mdr input; visual_err input
function F = fcn(Pos_pr,V_pr,Pos_dr,V_dr,Mdr,visual_err)
% 在x方向，椎管刚接触到锥套的时候，两者差是0.2m，完全进入时两者差是0.8
% 在z方向，椎管在锥套最下沿的时候，两者差是0.21m，在正中间的时候是0.12m 感觉这个不准
% error =z^2+y^2-x^2; 
% error<0 代表在圆锥里面
% 当x进入一定范围之内时，才能计算误差
% 当前位置减去定点的位置 相当于把定点放在了原点 x^2 = y^2 + z^2 （x<0）
% 分成xyz三个方向进行误差计算 
% x的范围[-0.2,0.45]  yz的范围相同,就是x一定时，半径时y=z=x对应的圆形的范围[-y,y]
% 给定了x之后 要判断两个 第一个是在这个圆形范围内，第二个是距离圆心的距
F = zeros(3,1);
% modify = [0.66;-0.1;0.645]*0+[0.7;-0.1;0.8]*0;
modify = visual_err;
% 是锥套位置-椎管位置 初始值是大于0的
x = Pos_dr(1) - Pos_pr(1)+ modify(1);
y = Pos_dr(2) - Pos_pr(2)+ modify(2);
% 椎管的z坐标要反一下 
z = Pos_dr(3) - Pos_pr(3)+ modify(3);
Vel_relative = V_pr - V_dr;

error =z^2+y^2-x^2; 
Kp_p = 100;
Kp_v = 50; 
persistent f;     
if(isempty(f))
    f=[0;0;0];
end
if x<0.05
%     F(1)= 1000 * Mdr * (-x) + 500 * Mdr * (Vel_relative(1));
%     % y方向的
%     F(2)= 1000 * Mdr * (-y) + 500 * Mdr * (Vel_relative(2));
%     % z方向的
%     F(3)= 1500 * Mdr * (-z) + 500 * Mdr * (Vel_relative(3));
    if x>-0.05
    F(1)= 100 * Mdr * (-x) + 1 * Mdr * (Vel_relative(1));
    % y方向的
    F(2)= 20 * Mdr * (-y) + 2 * Mdr * (Vel_relative(2));
    % z方向的
    F(3)= 20 * Mdr * (-z) + 2 * Mdr * (Vel_relative(3));
    f = F;
    else
        F=f;
    end
end
% F = zeros(3,1);

== matlab function AirRefueling_Platform_Varyingmass/Hose-drogue system/MATLAB Function ==
  data: P_dr input; P_link10 input; P_hose_dr output
function P_hose_dr = fcn(P_dr,P_link10)
% P_link20=zeros(3,20);
% P_link20(:,1) = P_link10(:,1)/2;
% P_link20(:,2) = P_link10(:,1);
% P_link20(:,3) = (P_link10(:,2)+P_link10(:,1))/2;
% P_link20(:,4) = P_link10(:,2);
% P_link20(:,5) = (P_link10(:,3)+P_link10(:,2))/2;
% P_link20(:,6) = P_link10(:,3);
% P_link20(:,7) = (P_link10(:,4)+P_link10(:,3))/2;
% P_link20(:,8) = P_link10(:,4);
% P_link20(:,9) = (P_link10(:,5)+P_link10(:,4))/2;
% P_link20(:,10) = P_link10(:,5);
% P_link20(:,11) = (P_link10(:,6)+P_link10(:,5))/2;
% P_link20(:,12) = P_link10(:,6);
% P_link20(:,13) = (P_link10(:,7)+P_link10(:,6))/2;
% P_link20(:,14) = P_link10(:,7);
% P_link20(:,15) = (P_link10(:,8)+P_link10(:,7))/2;
% P_link20(:,16) = P_link10(:,8);
% P_link20(:,17) = (P_link10(:,9)+P_link10(:,8))/2;
% P_link20(:,18) = P_link10(:,9);
% P_link20(:,19) = (P_link10(:,10)+P_link10(:,9))/2;
% P_link20(:,20) = P_link10(:,10);
% %P_link20(:,20) = P_dr;
% P_link20_V60 = reshape(P_link20,60,1);


%% 

x = P_link10(1,:);
y = P_link10(2,:);
z = P_link10(3,:);
n=length(x)-1;% B样条曲线有n+1个控制点
k=4;% 三次B样条，因此阶数=次数+1

% 用于储存生成的点
X=[];
Y=[];
Z=[];

Nik_u=zeros(1,n+1);% 用于储存基函数
nodevector=U_quasi_uniform(n,k);% 生成节点向量

for u=0:0.01:1-0.01% 循环次数决定组成B样条曲线点的总数量
    for j=1:n+1% 生成Bi,3这一系列基函数
        Nik_u(j)=BaseFunction(j,k,u,nodevector);
    end
    % 由于B样条曲线具有局部支撑性，因此只有u周围一定区间会参与到计算
    X=[X,x*Nik_u'];
    Y=[Y,y*Nik_u'];
    Z=[Z,z*Nik_u'];
end
% 根据三次B样条插值的结果得到20根管子的位置
P_link20=zeros(3,20);
index = 1;
for i=1:length(X)/20:100
    P_link20(:,index)=[X(i),Y(i),Z(i)];
    index = index+1;
end

P_link20_V60 = reshape(P_link20,60,1);
% 再将锥套的真实位置传过去 此时是63*1(20根管子+1个锥套)的向量 前面60个是软管 最后三个是锥套
P_hose_dr = [P_link20_V60;P_dr];

== matlab function AirRefueling_Platform_Varyingmass/Receiver system/F16 Nonlinear Model/constant mass model/pri_sys_controller/MATLAB Function ==
  settings: updateMethod=DISCRETE
  data: y output; t input
function y = fcn(t)

persistent tt;
if(isempty(tt))
  tt=0;
end

t1 = t-tt;
% if t1 < 10
%     xx = 0;
% elseif  t1 >= 10 && t1 < 70
%     xx = 50*sin(0.025*(t1-10));
% elseif  t1 >= 70 && t1 < 90
%     xx = 50;
% elseif  t1 >= 90 && t1 < 150
%     xx = 50-15*sin(0.025*(t1-90));
% else
%     xx = 35;
% end

% if t1 < 10
%     xx = 0;
% elseif  t1 >= 10 && t1 < 70
%     xx = 1*sin(0.025*(t1-10));
% else
%     xx = 1;
% end
xx = 0;

zz = 0;

y = [xx;zz];

end

== matlab function AirRefueling_Platform_Varyingmass/Receiver system/F16 Nonlinear Model/constant mass model/pri_sys_controller/MATLAB Function1 ==
  settings: updateMethod=DISCRETE
  data: y output; t input
function y = fcn(t)

persistent tt;
if(isempty(tt))
  tt=0;
end

t1 = t-tt;

% if t1 < 90
%     yy = 0;
% elseif  t1 >= 90 && t1 < 150
%     yy = 50*sin(0.025*(t1-90));
% else
%     yy = 50;
% end
% end

yy = 0;
y = yy;

== matlab function AirRefueling_Platform_Varyingmass/Receiver system/F16 Nonlinear Model/constant mass model/pri_sys_controller/MATLAB Function3 ==
  data: u input; y output
function y = fcn(u)

y = u([1,3,5,7,8,11]);

== matlab function AirRefueling_Platform_Varyingmass/Hose-drogue system/DRdynamics/Hose-Drogue1/Calculate the External Force of the Links/MATLAB Function ==
  data: vr input; n input; Ref output; radius input; viscosity input; Cf output; Red output; Cd output; N parameter
function [Ref, Cf, Red, Cd] = C(vr,n,radius,viscosity, N)
% 计算雷诺数以及相应的摩擦系数Cf和压差系数Cd

% 单杆的速度、方向等用3*1的列向量表示
% vr = 连杆相对风速度 向量3*N
% n = 连杆的方向向量，想上为正 向量3*N
% viscosity  = 动粘度系数
% radius = 连杆半径

%——计算雷诺数———————————————————————————
cosa = zeros(1,N);
sina = zeros(1,N);
Ref = zeros(1,N);
Red = zeros(1,N);
for i = 1:N
    if norm(vr(:,i)) ~= 0
        cosa(i) = vr(:,i)'*n(:,i)/norm(vr(:,i));
        sina(i) = sqrt(1-cosa(i)^2);
        if sina(i) ~= 0
            Ref(i) = (pi*radius/viscosity)*norm(vr(:,i))/sina(i);
        else
            Ref(i) = 10^11;
        end
        Red(i) = norm(vr(:,i))*2*radius/viscosity;
    end
end

%——计算气动系数——————————————————————————
Cf = zeros(1,N);
Cd = zeros(1,N);
for i = 1:N
    %%%%Cf表%%%%%%%%%%%%%%%%%%%%%%%%
    if Ref(i)<=10^-2
        Cf(i) = 0;    %注意这里有改动
    elseif Ref(i)>10^-2 && Ref(i)<=10^4
        Cf(i) = 4.6409*Ref(i)^-0.6667;
    elseif Ref(i)>10^4 && Ref(i)<=10^10
        Cf(i) = 0.0464*Ref(i)^-0.1667;
    elseif Ref(i)>10^10
        Cf(i) = 0.001;
    end
    %%%%Cd表%%%%%%%%%%%%%%%%%%%%%%%%%
    if Red(i)<=10^-2
        Cd(i) = 0;   %注意这里有改动
    elseif Red(i)>10^-2 && Red(i)<=1
        Cd(i) = 10*Red(i)^-0.801;
    elseif Red(i)>1 && Red(i)<=180
        Cd(i) = 10*Red(i)^-0.4083;
    elseif Red(i)>180 && Red(i)<=4*10^5
        Cd(i) = 1.2;
    elseif Red(i)>4*10^5 && Red(i)<=4*10^6
        Cd(i) = 0.002128*Red(i)^0.3522;
    elseif Red(i)>4*10^6
        Cd(i) = 0.45;
    end
end

== matlab function AirRefueling_Platform_Varyingmass/Hose-drogue system/DRdynamics/Hose-Drogue1/Calculate the External Force of the Links/MATLAB Function1 ==
  data: vr input; Q output; n input; Cf input; Cd input; l1 input; density input; radius input; Rdr input; Cdr input; Mdr input; rou input; p input; Fb input; Df_mid output; Dd_mid output; Df output; Dd output; D output; Ddr output; N parameter; l0 parameter; fen_norm output; fen output
function [Q, Df_mid, Dd_mid, Df, Dd, D, Ddr, fen_norm, fen] = ExternalForce(vr,n,Cf,Cd,l1,density,radius,Rdr,Cdr,Mdr,rou,p,Fb, N,l0)

% 计算每根连杆的合外力

% 单杆的速度、方向等用3*1的列向量表示
% l = 每根连杆的长度，注意这里要做成变长的 向量
% vr = 连杆相对风速度 向量3*N
% n = 连杆的方向向量，想上为正 向量3*N
% viscosity  = 大气动粘度系数
% density = 大气密度
% radius = 连杆半径
% r_dr = 锥套伞冠半径
% rou = 连杆的线密度

% Cdr = 锥套的阻力系数
% Rdr = 锥套伞冠半径
% Mdr = 锥套质量

%——求气动力————————————————————————————
Df_mid = zeros(1,N);
Dd_mid = zeros(1,N);
Df = zeros(3,N);
Dd = zeros(3,N);
D = zeros(3,N);
vn = zeros(3,N);
for i = 1:N
    if i == 1
        Df_mid(i) = density*pi*radius*l1*Cf(i)*(vr(:,i)'*n(:,i))^2;
    else
        Df_mid(i) = density*pi*radius*l0*Cf(i)*(vr(:,i)'*n(:,i))^2;
    end
    if vr(:,i)'*n(:,i)>0   % 这里可能有符号问题，万一之后还是出现杂乱的情况，要注意这里
        Df(:,i) = Df_mid(i)*n(:,i);
    else
        Df(:,i) = - Df_mid(i)*n(:,i);
    end
    % 当杆的方向迎着风的时候，摩擦阻力延杆反向
    % 当杆的方向顺着风的时候，摩擦阻力延杆正向
    
    vn(:,i) = vr(:,i)-(vr(:,i)'*n(:,i))*n(:,i); 
    if i == 1
        if norm(vn(:,i)) ~= 0
            Dd_mid(i) = density*radius*l1*Cd(i)*norm(vn(:,i))^2;
            Dd(:,i) = - Dd_mid(i)*vn(:,i)/norm(vn(:,i));
        else
            Dd(:,i) = [0;0;0];
        end
    else
        if norm(vn(:,i)) ~= 0
            Dd_mid(i) = density*radius*l0*Cd(i)*norm(vn(:,i))^2;
            Dd(:,i) = - Dd_mid(i)*vn(:,i)/norm(vn(:,i));
        else
            Dd(:,i) = [0;0;0];
        end
    end
    % 无论连杆与相对速度的角度关系如何，压差阻力总是顺着风的方向的
        
    D(:,i) = Df(:,i) + Dd(:,i);
end

if vr(:,N)'*vr(:,N) ~= 0
    Ddr = - 1/2*density*vr(:,N)'*vr(:,N)*(pi*Rdr^2)*(Cdr)* vr(:,N)/norm(vr(:,N));
else
    Ddr = [0;0;0];
end
%%%%%%%%%%%%%%%%%%%%%%%%%%%%%%%%%%%%%%%%%%%%%%%%%%%%%%%%%%%%%%%%

% %%%%计算恢复力%%%%%%%%%%%%%%%%%%%%%%
do = 1; % 连杆外径
di = 0.84; % 连杆内径
E = 589.67; % 弹性系数 数量级可能有问题
K = E*pi/8*(do^4 - di^4);
fen_norm = zeros(1,N);
fen = zeros(3,N);
for i = 2:N-1
    n0mid = (p(:,i-1) - p(:,i+1))/norm(p(:,i-1) - p(:,i+1));
    if abs(norm(n(:,i-1)'*n(:,i))-1) ~= 0;
        gama1 = n(:,i-1)'*n0mid;
        gama2 = n(:,i)'*n0mid;
        if norm(gama1) >= 1
            gama1 = gama1/abs(gama1);
        end
        if norm(gama2) >= 1
            gama2 = gama2/abs(gama2);
        end
            
        fen_norm(i) = K*(acos(gama1) + acos(gama2))/norm(p(:,i-1) - p(:,i+1))^2;
        fen(:,i) = fen_norm(i)*((n(:,i)'*n0mid*n0mid - n(:,i))*1e3)/norm((n(:,i)'*n0mid*n0mid - n(:,i))*1e3);
    end
end
%%%%%%%%%%%%%%%%%%%%%%%%%%%%%%%%%%%%%%

% %%%%计算合外力%%%%%%%%%%%%%%%%%%%%%%?
% Q = zeros(3,N);
% for i = 1:N-1
%     Q(:,i) = [0;0;m*g] + 1/2*(D(:,i)+D(:,i+1));
% end
% Q(:,N) = [0;0;(m+Mdr)*g] + 1/2*D(:,N) + Ddr;
Q = zeros(3,N);
Q(:,1) = [0;0;l1*rou*9.8] + 1/2*(D(:,1)+D(:,2)) + fen(:,1);
for i = 2:N-1
    Q(:,i) = [0;0;l0*rou*9.8] + 1/2*(D(:,i)+D(:,i+1)) + fen(:,i);
end
Q(:,N) = [0;0;(l0/2*rou + Mdr)*9.8] + 1/2*D(:,N) + Ddr + Fb;        %注意最后一个节点的质量
% 这里删掉了锥套的受力（Bow wave），后面再处理
% %%%%%%%%%%%%%%%%%%%%%%%%%%%%%%%%

== matlab function AirRefueling_Platform_Varyingmass/Hose-drogue system/DRdynamics/Hose-Drogue1/Calculate the Orientation of the Links1/MATLAB Function ==
  data: nd1 output; nd2 output; theta1 input; n output; theta2 input; N parameter
function [nd1,nd2,n] = fcn(theta1,theta2, N)
% theta1,theta2 向量1*n
n = zeros(3,N);
nd1 = zeros(3,N);
nd2 = zeros(3,N);

for i = 1:N
    n(:,i) = [cos(theta1(i))*cos(theta2(i)); sin(theta2(i)); -sin(theta1(i))*cos(theta2(i))];
    nd1(:,i) = [-sin(theta1(i))*cos(theta2(i)); 0; -cos(theta1(i))*cos(theta2(i))];
    nd2(:,i) = [-cos(theta1(i))*sin(theta2(i)); cos(theta2(i)); sin(theta1(i))*sin(theta2(i))];
end

== matlab function AirRefueling_Platform_Varyingmass/Hose-drogue system/DRdynamics/Hose-Drogue1/Calculate the Orientation of the Links1/MATLAB Function4 ==
  data: a input; a0 input; nd1 input; nd2 input; dn input; dnd1 input; dnd2 input; dtheta1 input; dtheta2 input; l1 input size=1; dl1 input; ddtheta1 output; ddtheta2 output; N parameter; l0 parameter
function [ddtheta1,ddtheta2] = fcn(a,a0,nd1,nd2,dn,dnd1,dnd2,dtheta1,dtheta2,l1,dl1, N, l0)
% theta1,theta2 向量N*1
% omiga,alpha是加油机坐标系的旋转角速度和叫加速度
% a是各节点的加速度
% a0为加油机加速度
% l,dl,ddl是连杆的长度及其一二阶导数

ddtheta1 = zeros(1,N);
ddtheta2 = zeros(1,N);

ddtheta1(1) = nd1(:,1)'*(-(a(:,1)-a0)-2*dl1*dn(:,1)-...
              l1*(dnd1(:,1)*dtheta1(1)+dnd2(:,1)*dtheta2(1)))...
              /(l1*norm(nd1(:,1)));
ddtheta2(1) = nd2(:,1)'*(-(a(:,1)-a0)-2*dl1*dn(:,1)-...
              l1*(dnd1(:,1)*dtheta1(1)+dnd2(:,1)*dtheta2(1)))...
              /(l1*norm(nd2(:,1)));
for i = 2:N
    ddtheta1(i) = nd1(:,i)'*(-(a(:,i)-a(:,i-1))-...
                  l0*(dnd1(:,i)*dtheta1(i)+dnd2(:,i)*dtheta2(i)))...
                  /(l0*norm(nd1(:,i)));
    ddtheta2(i) = nd2(:,i)'*(-(a(:,i)-a(:,i-1))-...
                  l0*(dnd1(:,i)*dtheta1(i)+dnd2(:,i)*dtheta2(i)))...
                  /(l0*norm(nd2(:,i)));
end
